simulink model "pendule_inv_capteur_etu"  (R2022b)
settings: Solver=VariableStepAuto  StartTime=0.0  StopTime=10.0  RelTol=1e-3
values from neighbouring files (symbols this model uses):
  g = 9.81    [simu_pendule_inv_etu.m]
  K = [30 10]    [simu_pendule_inv_etu.m]
  l = 10    [simu_pendule_inv_etu.m]
  ue = 0    [simu_pendule_inv_etu.m]
  x0 = [pi/10 0]'    [simu_pendule_inv_etu.m]
  xe = [0 0]'    [simu_pendule_inv_etu.m]
settings Model: Creator=felix  LastModifiedBy=felix

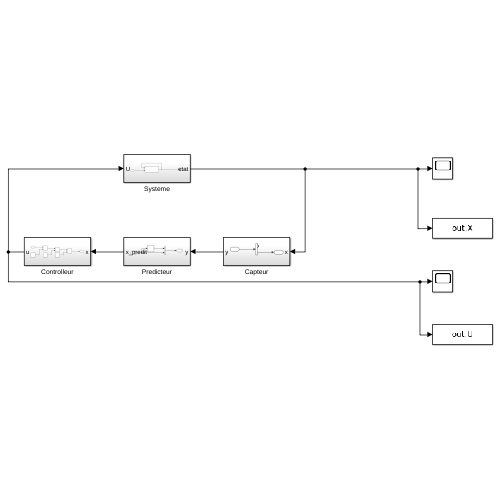
[thumbnail: Simulink's stored preview of the top-level diagram]
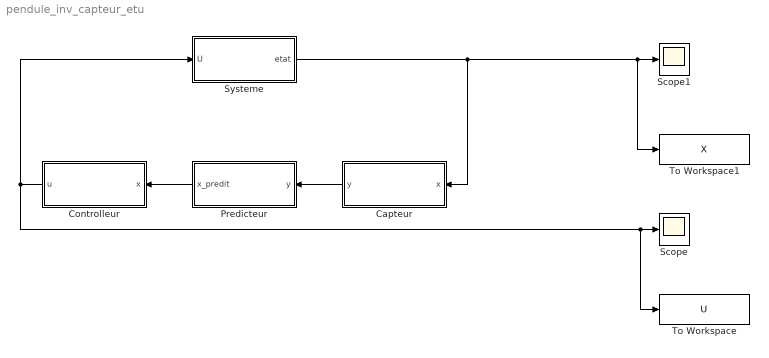
== system pendule_inv_capteur_etu ==
  Capteur : Subsystem
  Controlleur : Subsystem
  Predicteur : Subsystem
  Scope : Scope
  Scope1 : Scope
  Systeme : Subsystem
  To Workspace : ToWorkspace  VariableName=U  SaveFormat=Timeseries  SampleTime=-1
  To Workspace1 : ToWorkspace  VariableName=X  SaveFormat=Timeseries  SampleTime=-1
  wires:
  Capteur/1(y) -> Predicteur/1(y)
  Systeme/1(etat) -> Capteur/1(x), To Workspace1/1, Scope1/1
  Predicteur/1(x_predit) -> Controlleur/1(x)
  Controlleur/1(u) -> To Workspace/1, Scope/1, Systeme/1(U)

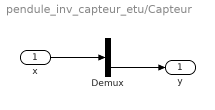
== system pendule_inv_capteur_etu/Capteur ==
  x : Inport
  Demux : Demux  Outputs=2
  y : Outport
  wires:
  x/1 -> Demux/1
  Demux/2 -> y/1

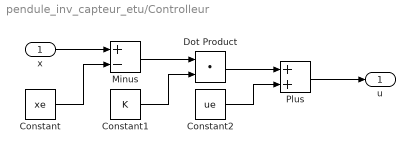
== system pendule_inv_capteur_etu/Controlleur ==
  x : Inport
  Constant : Constant  Value=xe
  Constant1 : Constant  Value=K
  Constant2 : Constant  Value=ue
  Dot Product : DotProduct  OutDataTypeStr=Inherit: Inherit via internal rule
  Minus : Sum  Inputs=+-
  Plus : Sum
  u : Outport
  wires:
  Minus/1 -> Dot Product/1
  Plus/1 -> u/1
  Constant/1 -> Minus/2
  Constant2/1 -> Plus/2
  Constant1/1 -> Dot Product/2
  x/1 -> Minus/1
  Dot Product/1 -> Plus/1

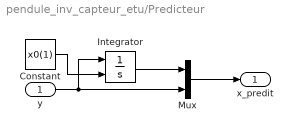
== system pendule_inv_capteur_etu/Predicteur ==
  y : Inport
  Constant : Constant  Value=x0(1)
  Integrator : Integrator  InitialConditionSource=external  InitialCondition=x0(1)
  Mux : Mux  Inputs=2
  x_predit : Outport
  wires:
  y/1 -> Integrator/1, Mux/2
  Integrator/1 -> Mux/1
  Mux/1 -> x_predit/1
  Constant/1 -> Integrator/2

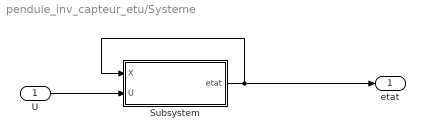
== system pendule_inv_capteur_etu/Systeme ==
  U : Inport
  Subsystem : Subsystem
  etat : Outport
  wires:
  U/1 -> Subsystem/2(U)
  Subsystem/1(etat) -> Subsystem/1(X), etat/1

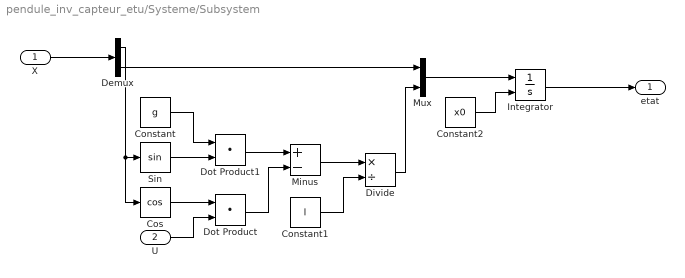
== system pendule_inv_capteur_etu/Systeme/Subsystem ==
  X : Inport
  U : Inport  Port=2
  Constant : Constant  Value=g
  Constant1 : Constant  Value=l
  Constant2 : Constant  Value=x0
  Cos : Trigonometry  Operator=cos
  Demux : Demux  Outputs=2
  Divide : Product  Inputs=*/  RndMeth=Zero  SaturateOnIntegerOverflow=on
  Dot Product : DotProduct  OutDataTypeStr=Inherit: Inherit via internal rule
  Dot Product1 : DotProduct  OutDataTypeStr=Inherit: Inherit via internal rule
  Integrator : Integrator  InitialConditionSource=external
  Minus : Sum  Inputs=+-
  Mux : Mux  Inputs=2
  Sin : Trigonometry
  etat : Outport
  wires:
  X/1 -> Demux/1
  Mux/1 -> Integrator/1
  Demux/2 -> Mux/1
  Integrator/1 -> etat/1
  Demux/1 -> Cos/1, Sin/1
  Cos/1 -> Dot Product/1
  U/1 -> Dot Product/2
  Sin/1 -> Dot Product1/2
  Constant/1 -> Dot Product1/1
  Dot Product1/1 -> Minus/1
  Dot Product/1 -> Minus/2
  Minus/1 -> Divide/1
  Constant1/1 -> Divide/2
  Divide/1 -> Mux/2
  Constant2/1 -> Integrator/2
